simulink model "SimulinkDuhemModel"  (R2020a)
settings: Solver=ode4  StartTime=0.0  StopTime=10  FixedStep=1e-6  RelTol=1e-3  EnableMultiTasking=on
values from neighbouring files (symbols this model uses):
  amp = 15    [SimulinkCreateParams.m]
  bias = 0    [SimulinkCreateParams.m]
  freq = 2*pi/T    (= 3.14159265359)    [SimulinkCreateParams.m]
  phase = pi-asin(sign(u0)*min([abs(u0),amp])/amp)    [SimulinkCreateParams.m]
  y0 = -10    [SimulinkCreateParams.m]
undefined symbols (not defined in the file or in its folder): curve1, curve2
libraries: simulink x1
settings Model: Creator=P255568  LastModifiedBy=M. Vasquez Beltran
settings DataIOCC: SaveFormat=Array  SignalLoggingSaveFormat=ModelDataLogs  ReturnWorkspaceOutputs=off
settings OptimizationCC: ExpressionDepthLimit=2147483647  InitFltsAndDblsToZero=on  LifeSpan=inf
settings DebuggingCC: UnderspecifiedInitializationDetection=Classic  MergeDetectMultiDrivingBlocksExec=none  SolverPrmCheckMsg=warning  FcnCallInpInsideContextMsg=warning  StateNameClashWarn=warning  SFUnexpectedBacktrackingDiag=warning  SFNoUnconditionalDefaultTransitionDiag=warning  SFExecutionAtInitializationDiag=none  ArithmeticOperatorsInVariantConditions=warning
settings HardwareCC: ProdBitPerPointer=32  ProdBitPerSizeT=32  ProdBitPerPtrDiffT=32  ProdLargestAtomicFloat=None  ProdIntDivRoundTo=Undefined  ProdEndianess=Unspecified  ProdWordSize=32  ProdHWDeviceType=32-bit Generic
settings ModelReferenceCC: PropagateSignalLabelsOutOfModel=off
settings SFSimCC: SimUseLocalCustomCode=off  CustomCodeUndefinedFunction=UseInterfaceOnly
settings RTWCC: RTWUseLocalCustomCode=off
settings CodeAppCC: StateflowObjectComments=on
settings GRTTargetCC: TargetLangStandard=C89/C90 (ANSI)  CombineOutputUpdateFcns=off  GRTInterface=on
settings ConfigComp: CovMetricSettings=dw  CovHtmlReporting=on  CovSaveCumulativeToWorkspaceVar=on  CovSaveSingleToWorkspaceVar=on  CovExternalEMLEnable=off

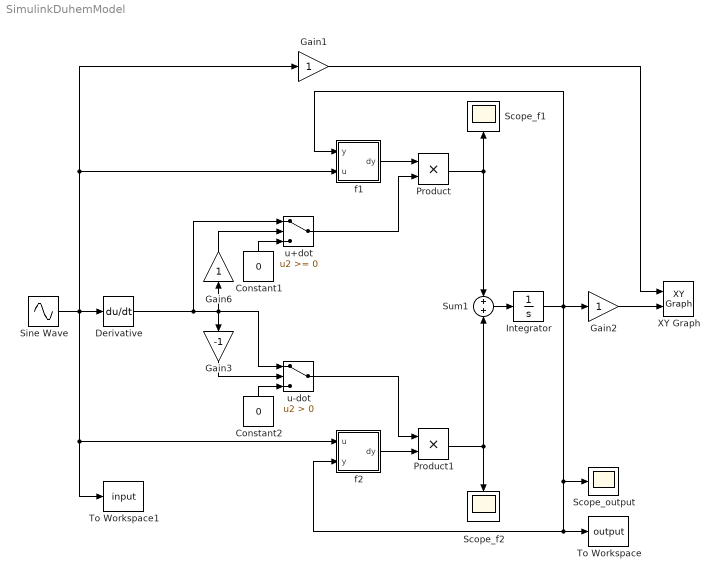
== system SimulinkDuhemModel ==
  Constant1 : Constant  Value=0
  Constant2 : Constant  Value=0
  Derivative : Derivative
  Gain1 : Gain
  Gain2 : Gain
  Gain3 : Gain  Gain=-1
  Gain6 : Gain
  Integrator : Integrator  InitialCondition=y0
  Product : Product  RndMeth=Zero
  Product1 : Product  RndMeth=Zero
  Scope_f1 : Scope
  Scope_f2 : Scope
  Scope_output : Scope
  Sine Wave : Sin  Amplitude=amp  Bias=bias  Frequency=freq  Phase=phase  SampleTime=0
  Sum1 : Sum  Inputs=+|+
  To Workspace : ToWorkspace  VariableName=output  SaveFormat=Timeseries  SampleTime=-1
  To Workspace1 : ToWorkspace  VariableName=input  SaveFormat=Timeseries  SampleTime=-1
  XY Graph : simulink/Sinks/XY Graph  xmin=xMin  xmax=xMax  ymin=yMin  ymax=yMax  st=-1
  f1 : MATLAB Function  TreatAsAtomicUnit=on
  f2 : MATLAB Function  TreatAsAtomicUnit=on
  u+dot : Switch
  u-dot : Switch  Criteria=u2 > Threshold
  wires:
  Sine Wave/1 -> f2/1(u), To Workspace1/1, f1/2(u), Gain1/1, Derivative/1
  Derivative/1 -> Gain3/1, Gain6/1, u-dot/1, u+dot/1
  Constant1/1 -> u+dot/3
  Gain3/1 -> u-dot/2
  Constant2/1 -> u-dot/3
  Gain6/1 -> u+dot/2
  f2/1(dy) -> Product1/2
  u-dot/1 -> Product1/1
  f1/1(dy) -> Product/1
  u+dot/1 -> Product/2
  Sum1/1 -> Integrator/1
  Product1/1 -> Scope_f2/1, Sum1/2
  Product/1 -> Scope_f1/1, Sum1/1
  Integrator/1 -> f1/1(y), f2/2(y), To Workspace/1, Scope_output/1, Gain2/1
  Gain1/1 -> XY Graph/1
  Gain2/1 -> XY Graph/2

== matlab function SimulinkDuhemModel/f2 ==
  data: u input; y input; curve1 parameter; curve2 parameter; dy output
function dy = f2(u,y,curve1,curve2)

point=[u,y];

%% Harcoded values
% scale = 2.0;
% if(ButterflyUtils.verticalDistance(point,curveAnhys)<=0)
%     if(ButterflyUtils.horizonalDistance(point,curve2)>0)
%         dy = 1.0*scale;
%     elseif(ButterflyUtils.horizonalDistance(point,curve1)>=0)
%         dy = -1.0*scale;
%     else
%         dy = -2.0*scale;
%     end
% else
%     if(ButterflyUtils.horizonalDistance(point,curve1)>0)
%         dy = 2.0*scale;
%     elseif(ButterflyUtils.horizonalDistance(point,curve2)>=0)
%         dy = 1.0*scale;
%     else
%         dy = -1.0*scale;
%     end
% end

%% Distance f2
% dy = -ButterflyUtils.signedClosestDistance(point,curve2);

% dy = ButterflyUtils.verticalDistance(point,curve2);

% dy = 0.05*ButterflyUtils.horizonalDistance(point,curve2);
% if(dy<0) dy=dy*10; end;

% dy = -ButterflyUtils.verticalDistance(point,curve1);

%% Bouc-wen f2
bw_alpha = 1;
bw_beta = 2;
bw_zeta = 1;
bw_n = 3;
dy = bw_alpha ...
        - bw_beta*abs(y)^bw_n ...
        + bw_zeta*y*abs(y)^(bw_n-1);
end

== matlab function SimulinkDuhemModel/f1 ==
  data: y input; u input; dy output; curve1 parameter; curve2 parameter
function dy = f1(y,u,curve1,curve2)

point=[u,y];

%% Harcoded values
% scale = 2.0;
% if(ButterflyUtils.verticalDistance(point,curveAnhys)<=0)
%     if(ButterflyUtils.horizonalDistance(point,curve2)>0)
%         dy = 2.0*scale;
%     elseif(ButterflyUtils.horizonalDistance(point,curve1)>=0)
%         dy = 1.0*scale;
%     else
%         dy = -1.0*scale;
%     end
% else
%     if(ButterflyUtils.horizonalDistance(point,curve1)>0)
%         dy = 1.0*scale;
%     elseif(ButterflyUtils.horizonalDistance(point,curve2)>=0)
%         dy = -1.0*scale;
%     else
%         dy = -2.0*scale;
%     end
% end

%% Distance f1
% dy = ButterflyUtils.signedClosestDistance(point,curve1);

% dy = -ButterflyUtils.verticalDistance(point,curve1);

% dy = -0.05*ButterflyUtils.horizonalDistance(point,curve1);
% if(dy>0) dy=dy*10; end;

% dy = -ButterflyUtils.verticalDistance(point,curve2);

%% Bouc-wen f1
bw_alpha = 1;
bw_beta = 2;
bw_zeta = 1;
bw_n = 3;
dy = bw_alpha ...
        - bw_beta*abs(y)^bw_n ...
        - bw_zeta*y*abs(y)^(bw_n-1);

end
